simulink model "model"  (R2023b)
settings: Solver=VariableStepAuto  StartTime=0.0  StopTime=30  MaxStep=1e-4  RelTol=1e-3
values from neighbouring files (symbols this model uses):
  bp = 5e-5    (= 5e-05)    [data.m]
  br = 1e-3    (= 0.001)    [data.m]
  g = 9.81    [data.m]
  Jp = mp*Lp^2/3    (= 0.000133128)    [data.m]
  Jr = mr*r^2/3    (= 0.000228791666667)    [data.m]
  km = kt    (= 0.042)    [data.m]
  kt = 0.042    [data.m]
  l = Lp/2    (= 0.0645)    [data.m]
  mp = 0.024    [data.m]
  r = 0.085    [data.m]
  Rm = 9.7    [data.m]
undefined symbols (not defined in the file or in its folder): ic_alpha0
libraries: simulink_extras x2
settings Model: Creator=renzo  LastModifiedBy=renzo

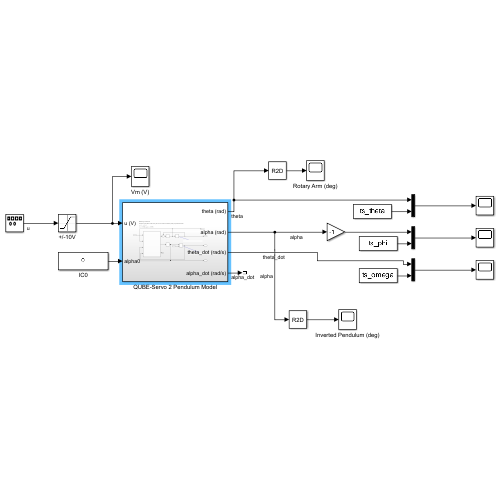
[thumbnail: Simulink's stored preview of the top-level diagram]
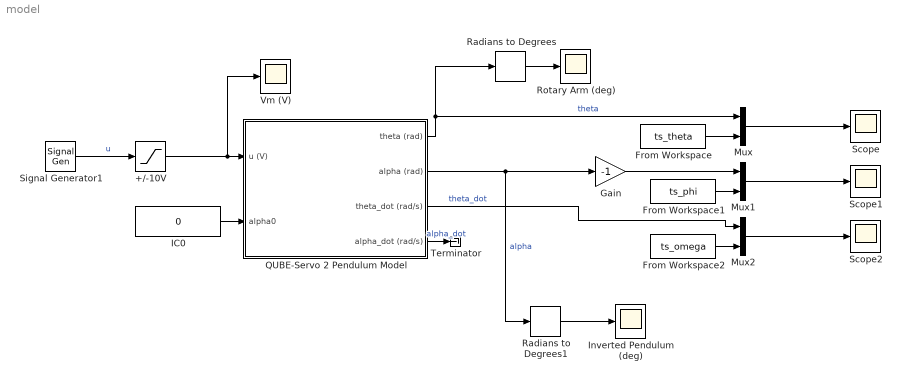
== system model ==
  +/-10V : Saturate  UpperLimit=10  LowerLimit=-10  OutDataTypeStr=Inherit: Inherit via back propagation
  From Workspace : FromWorkspace  VariableName=ts_theta
  From Workspace1 : FromWorkspace  VariableName=ts_phi
  From Workspace2 : FromWorkspace  VariableName=ts_omega
  Gain : Gain  Gain=-1
  IC0 : Constant  Value=0
  Inverted Pendulum (deg) : Scope
  Mux : Mux  Inputs=2
  Mux1 : Mux  Inputs=2
  Mux2 : Mux  Inputs=2
  QUBE-Servo 2 Pendulum Model : Subsystem
  Radians to Degrees : simulink_extras/Transformations/Radians to Degrees
  Radians to Degrees1 : simulink_extras/Transformations/Radians to Degrees
  Rotary Arm (deg) : Scope
  Scope : Scope
  Scope1 : Scope
  Scope2 : Scope
  Signal Generator1 : SignalGenerator  WaveForm=square  Amplitude=0.5  Frequency=0.5
  Terminator : Terminator
  Vm (V) : Scope
  wires:
  IC0/1 -> QUBE-Servo 2 Pendulum Model/2(alpha0)
  Radians to Degrees1/1 -> Inverted Pendulum (deg)/1
  +/-10V/1 -> QUBE-Servo 2 Pendulum Model/1(u (V)), Vm (V)/1
  QUBE-Servo 2 Pendulum Model/2(alpha (rad)) -> Gain/1, Radians to Degrees1/1  "alpha"
  QUBE-Servo 2 Pendulum Model/1(theta (rad)) -> Mux/1, Radians to Degrees/1  "theta"
  Signal Generator1/1 -> +/-10V/1  "u"
  Radians to Degrees/1 -> Rotary Arm (deg)/1
  QUBE-Servo 2 Pendulum Model/3(theta_dot (rad/s)) -> Mux2/1  "theta_dot"
  Mux2/1 -> Scope2/1
  From Workspace2/1 -> Mux2/2
  Mux/1 -> Scope/1
  From Workspace1/1 -> Mux1/2
  Mux1/1 -> Scope1/1
  From Workspace/1 -> Mux/2
  QUBE-Servo 2 Pendulum Model/4(alpha_dot (rad/s)) -> Terminator/1  "alpha_dot"
  Gain/1 -> Mux1/1

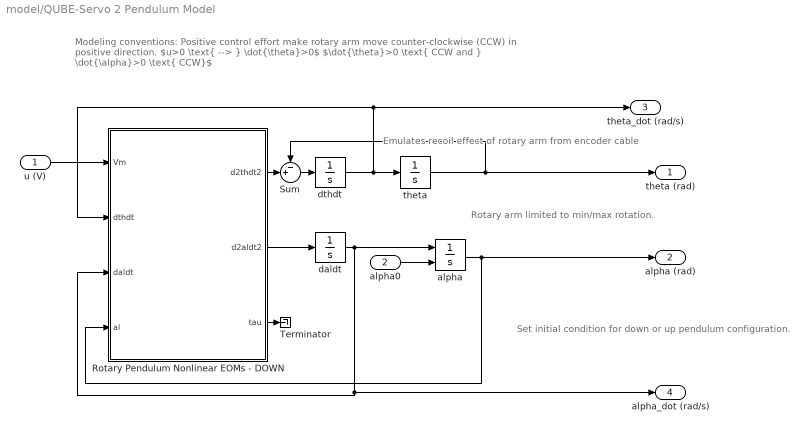
== system model/QUBE-Servo 2 Pendulum Model ==
  note: Rotary arm limited to min/max rotation.
  note: Modeling conventions:
      | Positive control effort make rotary arm move counter-clockwise (CCW) in positive direction.
      | $u>0 \text{ --> } \dot{\theta}>0$
      | $\dot{\theta}>0 \text{ CCW and } \dot{\alpha}>0 \text{ CCW}$
  note: Set initial condition for down or up pendulum configuration.
  note: Emulates recoil effect of rotary arm from encoder cable
  u (V) : Inport
  alpha0 : Inport  Port=2
  Rotary Pendulum Nonlinear EOMs - DOWN : MATLAB Function  TreatAsAtomicUnit=on
  Sum : Sum  Inputs=-+|
  Terminator : Terminator
  alpha : Integrator  InitialConditionSource=external  InitialCondition=ic_alpha0
  daldt : Integrator
  dthdt : Integrator
  theta : Integrator  LimitOutput=on  UpperSaturationLimit=2/3*pi  LowerSaturationLimit=-2/3*pi
  theta (rad) : Outport  VectorParamsAs1DForOutWhenUnconnected=off
  alpha (rad) : Outport  Port=2  VectorParamsAs1DForOutWhenUnconnected=off
  theta_dot (rad/s) : Outport  Port=3  VectorParamsAs1DForOutWhenUnconnected=off
  alpha_dot (rad/s) : Outport  Port=4  VectorParamsAs1DForOutWhenUnconnected=off
  wires:
  daldt/1 -> Rotary Pendulum Nonlinear EOMs - DOWN/3(daldt), alpha_dot (rad/s)/1, alpha/1
  Rotary Pendulum Nonlinear EOMs - DOWN/2(d2aldt2) -> daldt/1
  dthdt/1 -> theta_dot (rad/s)/1, Rotary Pendulum Nonlinear EOMs - DOWN/2(dthdt), theta/1
  u (V)/1 -> Rotary Pendulum Nonlinear EOMs - DOWN/1(Vm)
  Rotary Pendulum Nonlinear EOMs - DOWN/3(tau) -> Terminator/1
  alpha/1 -> alpha (rad)/1, Rotary Pendulum Nonlinear EOMs - DOWN/4(al)
  alpha0/1 -> alpha/2
  theta/1 -> theta (rad)/1, Sum/1
  Rotary Pendulum Nonlinear EOMs - DOWN/1(d2thdt2) -> Sum/2
  Sum/1 -> dthdt/1

== matlab function model/QUBE-Servo 2 Pendulum Model/Rotary Pendulum Nonlinear EOMs - DOWN ==
  data: Vm input size=1; d2thdt2 output size=1; d2aldt2 output size=1; dthdt input size=1; daldt input size=1; Jp parameter; Jr parameter; l parameter; mp parameter; br parameter; bp parameter; r parameter; kt parameter; km parameter; Rm parameter; al input size=1; g parameter; tau output
function [d2thdt2,d2aldt2,tau] = pen_nonlin_eoms(Vm, dthdt, daldt, Jp, Jr, l, mp, br, bp, r, kt, km, Rm, al, g)

% Convert voltage to torque input
tau = (Vm - km*dthdt)/Rm;
tau=kt*tau;
% Denominator
Jt = Jr*Jp + Jp^2*sin(al)^2 - mp^2*r^2*l^2*cos(al)^2;
% Nonlinear equations of motion for generic rotary pendulum (i.e. furuta)
% Terms from EOM solving
term1 = tau - br*dthdt + 2*Jp*sin(al)*cos(al)*dthdt*daldt + mp*r*l*sin(al)*daldt^2;
term2 = -bp*daldt - Jp*sin(al)*cos(al)*daldt^2 - mp*g*l*sin(al);
% Torque to rotary arm position)
d2thdt2 = 1/Jt*( Jp*term1 - mp*r*l*cos(al)*term2);
% Torque to pendulum angle position
d2aldt2 = 1/Jt*(-mp*r*l*cos(al)*term1 + (Jr+Jp*sin(al)^2)*term2);
